simulink model "regulation_singularity_free_TODO"  (R2025b)
settings: Solver=VariableStepAuto  StartTime=0.0  StopTime=10.0  RelTol=1e-3
values from neighbouring files (symbols this model uses):
  setpoints = dictionary()    [main.m]
undefined symbols (not defined in the file or in its folder): sim_trajectory_id
settings Model: Creator=Utente  LastModifiedBy=Utente

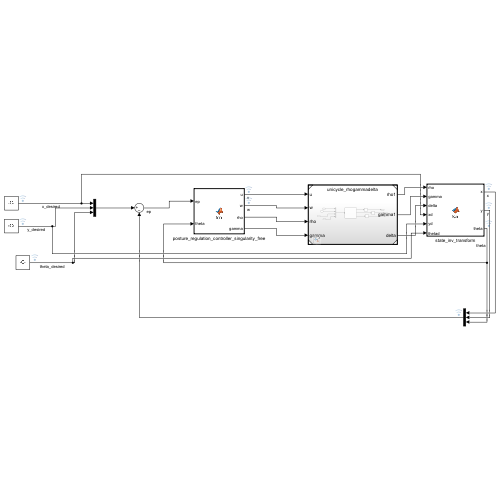
[thumbnail: Simulink's stored preview of the top-level diagram]
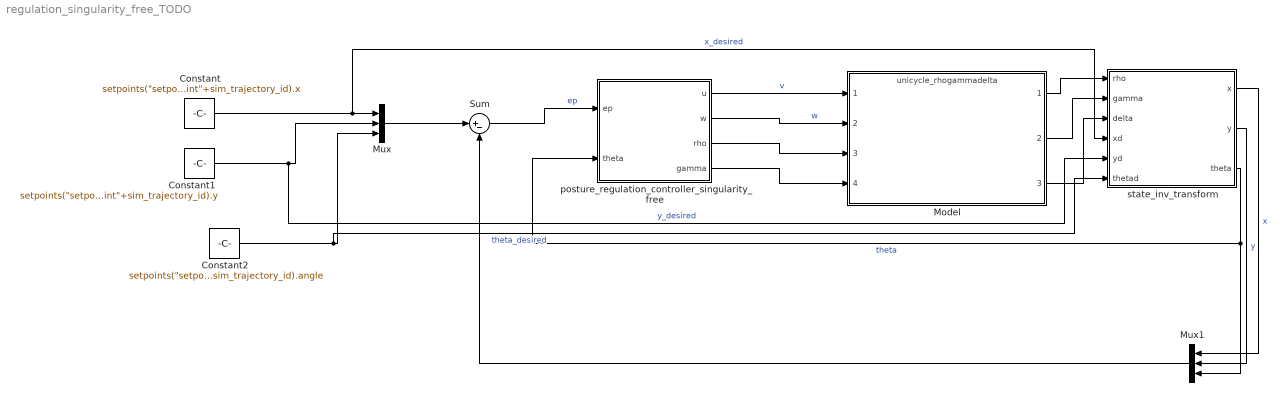
== system regulation_singularity_free_TODO ==
  Constant : Constant  Value="setpoints(\"setpoint\"+sim_trajectory_id).x"
  Constant1 : Constant  Value="setpoints(\"setpoint\"+sim_trajectory_id).y"
  Constant2 : Constant  Value="setpoints(\"setpoint\"+sim_trajectory_id).angle"
  Model : ModelReference  ModelNameDialog=unicycle_rhogammadelta.slx  SimulationMode=Normal  ModelReferenceVersion=1.2
  Mux : Mux  Inputs=3
  Mux1 : Mux  Inputs=3
  Sum : Sum  Inputs=|+-
  posture_regulation_controller_singularity_free : MATLAB Function  TreatAsAtomicUnit=on
  state_inv_transform : MATLAB Function  TreatAsAtomicUnit=on
  wires:
  Constant1/1 -> state_inv_transform/5(yd), Mux/2  "y_desired"
  Constant/1 -> state_inv_transform/4(xd), Mux/1  "x_desired"
  Sum/1 -> posture_regulation_controller_singularity_free/1(ep)  "ep"
  Mux/1 -> Sum/1
  Constant2/1 -> state_inv_transform/6(thetad), Mux/3  "theta_desired"
  Mux1/1 -> Sum/2
  posture_regulation_controller_singularity_free/1(u) -> Model/1  "v"
  posture_regulation_controller_singularity_free/2(w) -> Model/2  "w"
  Model/1 -> state_inv_transform/1(rho)
  Model/2 -> state_inv_transform/2(gamma)
  Model/3 -> state_inv_transform/3(delta)
  state_inv_transform/1(x) -> Mux1/1  "x"
  state_inv_transform/2(y) -> Mux1/2  "y"
  state_inv_transform/3(theta) -> posture_regulation_controller_singularity_free/2(theta), Mux1/3  "theta"
  posture_regulation_controller_singularity_free/3(rho) -> Model/3
  posture_regulation_controller_singularity_free/4(gamma) -> Model/4

== matlab function regulation_singularity_free_TODO/posture_regulation_controller_singularity_free ==
  data: ep input; u output; w output; theta input; rho output; gamma output
function [u, w, rho, gamma] = fcn(ep, theta)

dx = ep(1);
dy = ep(2);
dtheta = -ep(3);

rho   = sqrt(dx^2 + dy^2);
%alpha = wrapToPi(atan2(dy, dx) - theta); 
%beta  = wrapToPi(dtheta - alpha);
gamma = wrapToPi(atan2(dy, dx) - theta);
delta = wrapToPi(dtheta - gamma);

k1 = 1;%1
k2 = 4;%4
k3 = 1.5;%1.5

u = k1 * cos(gamma);
w = k2 * gamma + k1 * sin(gamma) * cos(gamma)/gamma * (gamma+k3*delta);


end

== matlab function regulation_singularity_free_TODO/state_inv_transform ==
  data: rho input; x output; y output; gamma input; delta input; theta output; xd input; yd input; thetad input
function [x,y,theta] = fcn(rho, gamma, delta, xd, yd, thetad)
x     = xd - rho*cos(thetad+2*gamma+delta);
y     = yd - rho*sin(thetad+2*gamma+delta);
theta = thetad+gamma+delta;
theta = wrapToPi(theta);
end
